simulink model "Lab7"  (R2023a)
settings: Solver=VariableStepAuto  StartTime=0.0  StopTime=20  FixedStep=0.0001  MaxStep=0.001  RelTol=1e-3
values from neighbouring files (symbols this model uses):
  A = [0, 1, 0 ... (first row only)    [init.m]
  B = [0 ... (first row only)    [init.m]
  b = 0.6    [init.m]
  C = [1, 0, 0]    [init.m]
  c = 12    [init.m]
  k = 5    [init.m]
  L = [200 ... (first row only)    [init.m]
  T1 = 0.05    [init.m]
  T2 = 0.4    [init.m]
settings Model: Creator=Алексей  LastModifiedBy=Алексей

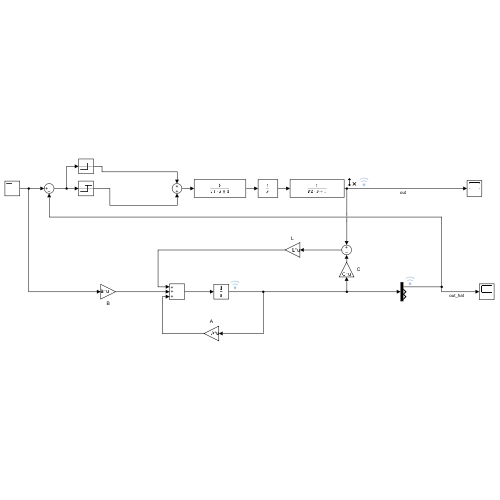
[thumbnail: Simulink's stored preview of the top-level diagram]
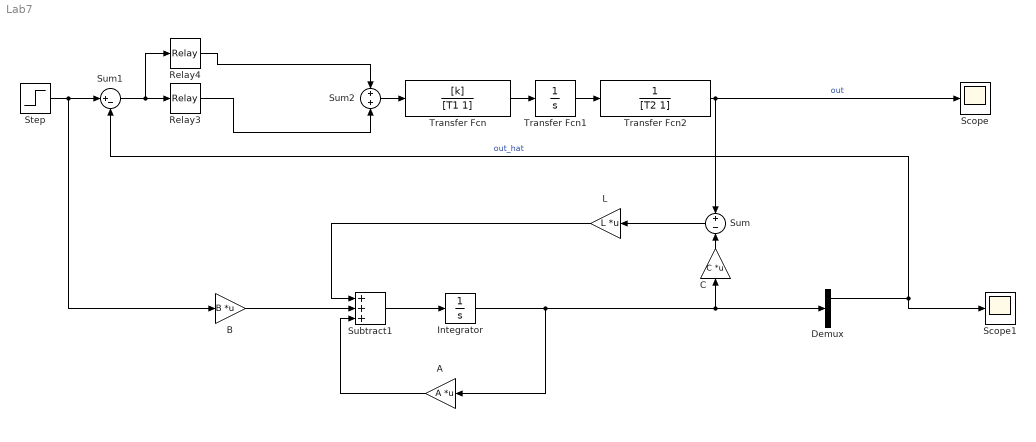
== system Lab7 ==
  A : Gain  Gain=A  Multiplication=Matrix(K*u)
  B : Gain  Gain=B  Multiplication=Matrix(K*u)
  C : Gain  Gain=C  Multiplication=Matrix(K*u)
  Demux : Demux  Outputs=3
  Integrator : Integrator
  L : Gain  Gain=L  Multiplication=Matrix(K*u)
  Relay3 : Relay  OnSwitchValue=b  OffSwitchValue=b  OnOutputValue=c  ZeroCross=off
  Relay4 : Relay  OnSwitchValue=-b  OffSwitchValue=-b  OnOutputValue=0  OffOutputValue=-c  ZeroCross=off
  Scope : Scope
  Scope1 : Scope
  Step : Step  Time=0.5  Before=1  After=0  SampleTime=0
  Subtract1 : Sum  Inputs=+++
  Sum : Sum  Inputs=+|-
  Sum1 : Sum  Inputs=|+-
  Sum2 : Sum  Inputs=+|+
  Transfer Fcn : TransferFcn  Numerator=[k]  Denominator=[T1 1]
  Transfer Fcn1 : TransferFcn  Denominator=[1 0]
  Transfer Fcn2 : TransferFcn  Denominator=[T2 1]
  wires:
  Relay3/1 -> Sum2/2
  Transfer Fcn/1 -> Transfer Fcn1/1
  Transfer Fcn1/1 -> Transfer Fcn2/1
  Relay4/1 -> Sum2/1
  Transfer Fcn2/1 -> Scope/1, Sum/1  "out"
  Subtract1/1 -> Integrator/1
  Integrator/1 -> Demux/1, C/1, A/1
  A/1 -> Subtract1/3
  Sum/1 -> L/1
  L/1 -> Subtract1/1
  C/1 -> Sum/2
  B/1 -> Subtract1/2
  Step/1 -> Sum1/1, B/1
  Demux/1 -> Scope1/1, Sum1/2  "out_hat"
  Sum1/1 -> Relay3/1, Relay4/1
  Sum2/1 -> Transfer Fcn/1
